simulink model "Perfiles"  (Simulink 8.5)
settings: Solver=ode45  StartTime=0.0  StopTime=tf  RelTol=1e-3
values from neighbouring files (symbols this model uses):
  Kp11 = 238.3924    [EtanolFouriergradiente.m]
  Kp12 = 35.9587    [EtanolFouriergradiente.m]
  Kp1I = 2.7378    [EtanolFouriergradiente.m]
  kp1I = 9.9722    [EtanolFouriergradiente.m]
  Ks1 = 159.7525    [EtanolFouriergradiente.m]
  Ks1I = 94.2332    [EtanolFouriergradiente.m]
  Ks1p1 = 1.3409    [EtanolFouriergradiente.m]
  ks1p1 = 18.6121    [EtanolFouriergradiente.m]
  Ks1p2 = 6.7116    [EtanolFouriergradiente.m]
  ks1p2 = 0.5863    [EtanolFouriergradiente.m]
  Ks2 = 0.0726    [EtanolFouriergradiente.m]
  Ks2I = 9.0048    [EtanolFouriergradiente.m]
  Ks2p1 = 0.9129    [EtanolFouriergradiente.m]
  ks2p1 = 1000    [EtanolFouriergradiente.m]
  Ks2p2 = 0.4310    (= 0.431)    [EtanolFouriergradiente.m]
  ks2p2 = 1.150    (= 1.15)    [EtanolFouriergradiente.m]
  landa = 0.5    [EtanolFouriergradiente.m]
  P10 = 5.3    [EtanolFouriergradiente.m]
  P20 = 0.0001    [EtanolFouriergradiente.m]
  S10 = 8.6    [EtanolFouriergradiente.m]
  S20 = 8.6    [EtanolFouriergradiente.m]
  Sf = 300    [EtanolFouriergradiente.m]
  T0 = 0.01    [EtanolFouriergradiente.m]
  um1 = 1.8823    [EtanolFouriergradiente.m]
  um2 = 1.7098    [EtanolFouriergradiente.m]
  V0 = 1.35    [EtanolFouriergradiente.m]
  vs1p1 = 1.5051    [EtanolFouriergradiente.m]
  vs1p2 = 0.00235    [EtanolFouriergradiente.m]
  vs2p1 = 0.3321    [EtanolFouriergradiente.m]
  vs2p2 = 0.1609    [EtanolFouriergradiente.m]
  X0 = 1.5    [EtanolFouriergradiente.m]
  Yp1s1 = 0.5085    [EtanolFouriergradiente.m]
  Yp1s2 = 0.5098    [EtanolFouriergradiente.m]
  Yp2s1 = 0.5331    [EtanolFouriergradiente.m]
  Yp2s2 = 0.4462    [EtanolFouriergradiente.m]
settings Model: Creator=CECI  LastModifiedBy=User
settings DebuggingCC: SolverPrmCheckMsg=warning  FcnCallInpInsideContextMsg=UseLocalSettings

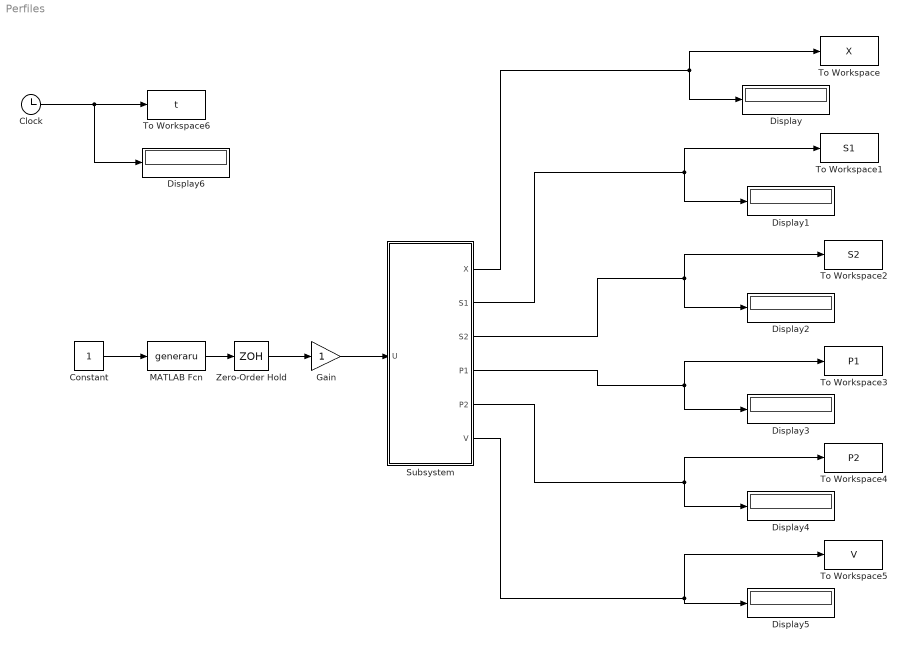
== system Perfiles ==
  Clock : Clock
  Constant : Constant
  Display{,1..6} (7 alike) : Display
  Gain : Gain
  MATLAB Fcn : MATLABFcn  MATLABFcn=generaru  SampleTime=T0
  Subsystem : Subsystem
  To Workspace : ToWorkspace  VariableName=X  SampleTime=T0
  To Workspace1 : ToWorkspace  VariableName=S1  SampleTime=T0
  To Workspace2 : ToWorkspace  VariableName=S2  SampleTime=T0
  To Workspace3 : ToWorkspace  VariableName=P1  SampleTime=T0
  To Workspace4 : ToWorkspace  VariableName=P2  SampleTime=T0
  To Workspace5 : ToWorkspace  VariableName=V  SampleTime=T0
  To Workspace6 : ToWorkspace  VariableName=t  SampleTime=T0
  Zero-Order Hold : ZeroOrderHold  SampleTime=T0
  wires:
  Subsystem/1(X) -> To Workspace/1, Display/1
  Subsystem/2(S1) -> To Workspace1/1, Display1/1
  Clock/1 -> To Workspace6/1, Display6/1
  MATLAB Fcn/1 -> Zero-Order Hold/1
  Constant/1 -> MATLAB Fcn/1
  Zero-Order Hold/1 -> Gain/1
  Gain/1 -> Subsystem/1(U)
  Subsystem/6(V) -> To Workspace5/1, Display5/1
  Subsystem/5(P2) -> Display4/1, To Workspace4/1
  Subsystem/3(S2) -> To Workspace2/1, Display2/1
  Subsystem/4(P1) -> To Workspace3/1, Display3/1

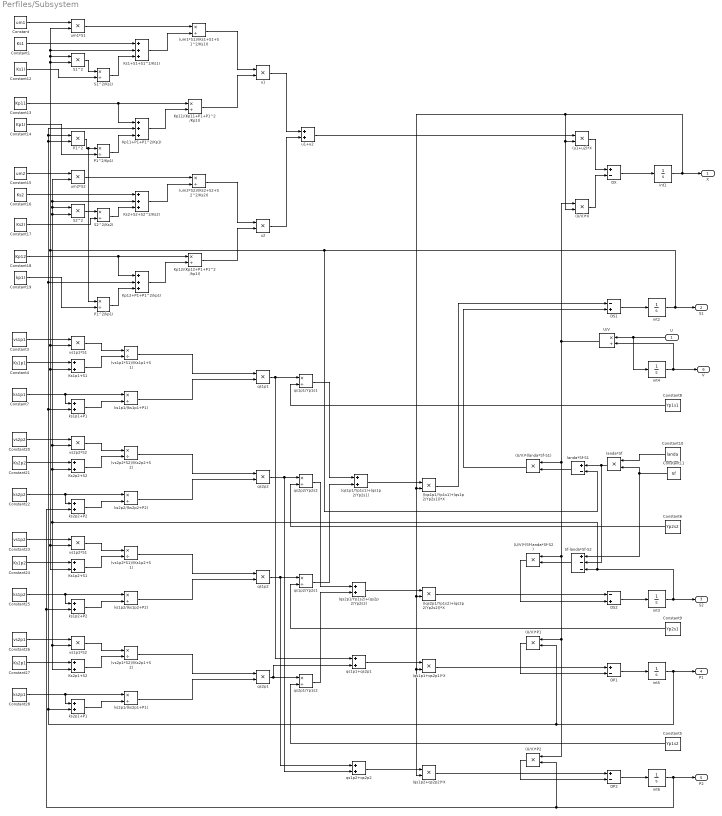
== system Perfiles/Subsystem ==
  U : Inport
  ((qs1p1/Yp1s1)+(qs1p2/Yp2s1))*X : Product  RndMeth=Zero
  ((qs2p1/Yp1s2)+(qs2p2/Yp2s2))*X : Product  RndMeth=Zero
  (U/V)*(Sf-landa*Sf-S2) : Product  RndMeth=Zero
  (U/V)*(landa*Sf-S1) : Product  RndMeth=Zero
  (U/V)*P1 : Product  RndMeth=Zero
  (U/V)*P2 : Product  RndMeth=Zero
  (U/V)*X : Product  RndMeth=Zero
  (qs1p1+qs2p1)*X : Product  RndMeth=Zero
  (qs1p1/Yp1s1)+(qs1p2/Yp2s1) : Sum
  (qs1p2+qs2p2)*X : Product  RndMeth=Zero
  (qs2p1/Yp1s2)+(qs2p2/Yp2s2) : Sum
  (u1+u2)*X : Product  RndMeth=Zero
  (um1*S1)/(Ks1+S1+S1^2/Ks1I) : Product  Inputs=*/
  (um2*S2)/(Ks2+S2+S2^2/Ks2I) : Product  Inputs=*/
  (vs1p1*S1)/(Ks1p1+S1) : Product  Inputs=*/
  (vs1p2*S1)/(Ks1p2+S1) : Product  Inputs=*/
  (vs2p1*S2)/(Ks2p1+S2) : Product  Inputs=*/
  (vs2p2*S2)/(Ks2p2+S2) : Product  Inputs=*/
  Constant : Constant  Value=um1
  Constant1 : Constant  Value=Ks1
  Constant10 : Constant  Value=landa
  Constant11 : Constant  Value=Sf
  Constant12 : Constant  Value=Ks1I
  Constant13 : Constant  Value=Kp11
  Constant14 : Constant  Value=Kp1I
  Constant15 : Constant  Value=um2
  Constant16 : Constant  Value=Ks2
  Constant17 : Constant  Value=Ks2I
  Constant18 : Constant  Value=Kp12
  Constant19 : Constant  Value=kp1I
  Constant20 : Constant  Value=vs2p2
  Constant21 : Constant  Value=Ks2p2
  Constant22 : Constant  Value=ks2p2
  Constant23 : Constant  Value=vs1p2
  Constant24 : Constant  Value=Ks1p2
  Constant25 : Constant  Value=ks1p2
  Constant26 : Constant  Value=vs2p1
  Constant27 : Constant  Value=Ks2p1
  Constant28 : Constant  Value=ks2p1
  Constant3 : Constant  Value=vs1p1
  Constant4 : Constant  Value=Ks1p1
  Constant5 : Constant  Value=Yp1s2
  Constant6 : Constant  Value=Yp2s2
  Constant7 : Constant  Value=ks1p1
  Constant8 : Constant  Value=Yp1s1
  Constant9 : Constant  Value=Yp2s1
  DP1 : Sum  Inputs=+-
  DP2 : Sum  Inputs=+-
  DS1 : Sum  Inputs=-+
  DS2 : Sum  Inputs=-+
  DX : Sum  Inputs=+-
  Kp11+P1+P1^2/Kp1I : Sum  Inputs=+++
  Kp11/(Kp11+P1+P1^2/Kp1I) : Product  Inputs=*/
  Kp12+P1+P1^2/kp1I : Sum  Inputs=+++
  Kp12/(Kp12+P1+P1^2/kp1I) : Product  Inputs=*/
  Ks1+S1+S1^2/Ks1I : Sum  Inputs=+++
  Ks1p1+S1 : Sum
  Ks1p2+S1 : Sum
  Ks2+S2+S2^2/Ks2I : Sum  Inputs=+++
  Ks2p1+S2 : Sum
  Ks2p2+S2 : Sum
  P1^2 : Product  RndMeth=Zero
  P1^2/Kp1I : Product  Inputs=*/
  P1^2/kp1I : Product  Inputs=*/
  S1^2 : Product  RndMeth=Zero
  S1^2/Ks1I : Product  Inputs=*/
  S2^2 : Product  RndMeth=Zero
  S2^2/Ks2I : Product  Inputs=*/
  Sf-landa*Sf-S2 : Sum  Inputs=+--
  U/V : Product  Inputs=*/
  int1 : Integrator  InitialCondition=X0  UpperSaturationLimit=40  LowerSaturationLimit=0
  int2 : Integrator  InitialCondition=S10  UpperSaturationLimit=10  LowerSaturationLimit=0
  int3 : Integrator  InitialCondition=S20  UpperSaturationLimit=100  LowerSaturationLimit=0
  int4 : Integrator  InitialCondition=V0  UpperSaturationLimit=10  LowerSaturationLimit=0
  int5 : Integrator  InitialCondition=P10  UpperSaturationLimit=100  LowerSaturationLimit=0
  int6 : Integrator  InitialCondition=P20  UpperSaturationLimit=100  LowerSaturationLimit=0
  ks1p1+P1 : Sum
  ks1p1/(ks1p1+P1) : Product  Inputs=*/
  ks1p2+P2 : Sum
  ks1p2/(ks1p2+P2) : Product  Inputs=*/
  ks2p1+P1 : Sum
  ks2p1/(ks2p1+P1) : Product  Inputs=*/
  ks2p2+P2 : Sum
  ks2p2/(ks2p2+P2) : Product  Inputs=*/
  landa*Sf : Product  RndMeth=Zero
  landa*Sf-S1 : Sum  Inputs=+-
  qs1p1 : Product  RndMeth=Zero
  qs1p1+qs2p1 : Sum
  qs1p1/Yp1s1 : Product  Inputs=*/
  qs1p2 : Product  RndMeth=Zero
  qs1p2+qs2p2 : Sum
  qs1p2/Yp2s1 : Product  Inputs=*/
  qs2p1 : Product  RndMeth=Zero
  qs2p1/Yp1s2 : Product  Inputs=*/
  qs2p2 : Product  RndMeth=Zero
  qs2p2/Yp2s2 : Product  Inputs=*/
  u1 : Product  RndMeth=Zero
  u1+u2 : Sum
  u2 : Product  RndMeth=Zero
  um1*S1 : Product  RndMeth=Zero
  um2*S2 : Product  RndMeth=Zero
  vs1p1*S1 : Product  RndMeth=Zero
  vs1p1*S2 : Product  RndMeth=Zero
  vs1p2*S1 : Product  RndMeth=Zero
  vs2p2*S2 : Product  RndMeth=Zero
  X : Outport
  S1 : Outport  Port=2
  S2 : Outport  Port=3
  P1 : Outport  Port=4
  P2 : Outport  Port=5
  V : Outport  Port=6
  wires:
  int1/1 -> X/1, (u1+u2)*X/2, (U/V)*X/2, ((qs1p1/Yp1s1)+(qs1p2/Yp2s1))*X/2, ((qs2p1/Yp1s2)+(qs2p2/Yp2s2))*X/2, (qs1p1+qs2p1)*X/2, (qs1p2+qs2p2)*X/2
  Constant/1 -> um1*S1/1
  S1^2/1 -> S1^2/Ks1I/1
  Constant12/1 -> S1^2/Ks1I/2
  Constant1/1 -> Ks1+S1+S1^2/Ks1I/1
  S1^2/Ks1I/1 -> Ks1+S1+S1^2/Ks1I/3
  P1^2/1 -> P1^2/Kp1I/1, P1^2/kp1I/1
  Constant14/1 -> P1^2/Kp1I/2
  P1^2/Kp1I/1 -> Kp11+P1+P1^2/Kp1I/3
  um1*S1/1 -> (um1*S1)/(Ks1+S1+S1^2/Ks1I)/1
  Ks1+S1+S1^2/Ks1I/1 -> (um1*S1)/(Ks1+S1+S1^2/Ks1I)/2
  Constant13/1 -> Kp11+P1+P1^2/Kp1I/1, Kp11/(Kp11+P1+P1^2/Kp1I)/1
  Kp11+P1+P1^2/Kp1I/1 -> Kp11/(Kp11+P1+P1^2/Kp1I)/2
  (um1*S1)/(Ks1+S1+S1^2/Ks1I)/1 -> u1/1
  Kp11/(Kp11+P1+P1^2/Kp1I)/1 -> u1/2
  Constant15/1 -> um2*S2/1
  S2^2/1 -> S2^2/Ks2I/1
  Constant17/1 -> S2^2/Ks2I/2
  Constant16/1 -> Ks2+S2+S2^2/Ks2I/1
  S2^2/Ks2I/1 -> Ks2+S2+S2^2/Ks2I/3
  Constant19/1 -> P1^2/kp1I/2
  P1^2/kp1I/1 -> Kp12+P1+P1^2/kp1I/3
  um2*S2/1 -> (um2*S2)/(Ks2+S2+S2^2/Ks2I)/1
  Ks2+S2+S2^2/Ks2I/1 -> (um2*S2)/(Ks2+S2+S2^2/Ks2I)/2
  Constant18/1 -> Kp12+P1+P1^2/kp1I/1, Kp12/(Kp12+P1+P1^2/kp1I)/1
  Kp12+P1+P1^2/kp1I/1 -> Kp12/(Kp12+P1+P1^2/kp1I)/2
  (um2*S2)/(Ks2+S2+S2^2/Ks2I)/1 -> u2/1
  Kp12/(Kp12+P1+P1^2/kp1I)/1 -> u2/2
  u1/1 -> u1+u2/1
  u2/1 -> u1+u2/2
  u1+u2/1 -> (u1+u2)*X/1
  (u1+u2)*X/1 -> DX/1
  (U/V)*X/1 -> DX/2
  DX/1 -> int1/1
  Constant3/1 -> vs1p1*S1/1
  Constant4/1 -> Ks1p1+S1/1
  vs1p1*S1/1 -> (vs1p1*S1)/(Ks1p1+S1)/1
  Ks1p1+S1/1 -> (vs1p1*S1)/(Ks1p1+S1)/2
  Constant7/1 -> ks1p1+P1/1, ks1p1/(ks1p1+P1)/1
  (vs1p1*S1)/(Ks1p1+S1)/1 -> qs1p1/1
  ks1p1/(ks1p1+P1)/1 -> qs1p1/2
  Constant20/1 -> vs2p2*S2/1
  Constant21/1 -> Ks2p2+S2/1
  vs2p2*S2/1 -> (vs2p2*S2)/(Ks2p2+S2)/1
  Ks2p2+S2/1 -> (vs2p2*S2)/(Ks2p2+S2)/2
  Constant22/1 -> ks2p2+P2/1, ks2p2/(ks2p2+P2)/1
  (vs2p2*S2)/(Ks2p2+S2)/1 -> qs2p2/1
  ks2p2/(ks2p2+P2)/1 -> qs2p2/2
  Constant23/1 -> vs1p2*S1/1
  Constant24/1 -> Ks1p2+S1/1
  vs1p2*S1/1 -> (vs1p2*S1)/(Ks1p2+S1)/1
  Ks1p2+S1/1 -> (vs1p2*S1)/(Ks1p2+S1)/2
  Constant25/1 -> ks1p2+P2/1, ks1p2/(ks1p2+P2)/1
  (vs1p2*S1)/(Ks1p2+S1)/1 -> qs1p2/1
  ks1p2/(ks1p2+P2)/1 -> qs1p2/2
  Constant26/1 -> vs1p1*S2/1
  Constant27/1 -> Ks2p1+S2/1
  vs1p1*S2/1 -> (vs2p1*S2)/(Ks2p1+S2)/1
  Ks2p1+S2/1 -> (vs2p1*S2)/(Ks2p1+S2)/2
  Constant28/1 -> ks2p1+P1/1, ks2p1/(ks2p1+P1)/1
  (vs2p1*S2)/(Ks2p1+S2)/1 -> qs2p1/1
  ks2p1/(ks2p1+P1)/1 -> qs2p1/2
  qs1p1/1 -> qs1p1/Yp1s1/1, qs1p1+qs2p1/1
  Constant8/1 -> qs1p1/Yp1s1/2
  qs1p2/1 -> qs1p2/Yp2s1/1, qs1p2+qs2p2/1
  Constant9/1 -> qs1p2/Yp2s1/2
  Constant6/1 -> qs2p2/Yp2s2/2
  qs2p2/1 -> qs2p2/Yp2s2/1, qs1p2+qs2p2/2
  qs2p1/1 -> qs2p1/Yp1s2/1, qs1p1+qs2p1/2
  Constant5/1 -> qs2p1/Yp1s2/2
  qs1p1/Yp1s1/1 -> (qs1p1/Yp1s1)+(qs1p2/Yp2s1)/1
  qs1p2/Yp2s1/1 -> (qs1p1/Yp1s1)+(qs1p2/Yp2s1)/2
  U/1 -> U/V/1, int4/1
  U/V/1 -> (U/V)*X/1, (U/V)*(landa*Sf-S1)/1, (U/V)*(Sf-landa*Sf-S2)/1, (U/V)*P1/1, (U/V)*P2/1
  (qs1p1/Yp1s1)+(qs1p2/Yp2s1)/1 -> ((qs1p1/Yp1s1)+(qs1p2/Yp2s1))*X/1
  Constant10/1 -> landa*Sf/1
  Constant11/1 -> landa*Sf/2, Sf-landa*Sf-S2/1
  landa*Sf/1 -> landa*Sf-S1/1, Sf-landa*Sf-S2/2
  landa*Sf-S1/1 -> (U/V)*(landa*Sf-S1)/2
  ((qs1p1/Yp1s1)+(qs1p2/Yp2s1))*X/1 -> DS1/1
  (U/V)*(landa*Sf-S1)/1 -> DS1/2
  int2/1 -> S1/1, landa*Sf-S1/2, S1^2/1, um1*S1/2, Ks1+S1+S1^2/Ks1I/2, S1^2/2, vs1p1*S1/2, Ks1p1+S1/2, vs1p2*S1/2, Ks1p2+S1/2
  DS1/1 -> int2/1
  qs2p1/Yp1s2/1 -> (qs2p1/Yp1s2)+(qs2p2/Yp2s2)/2
  qs2p2/Yp2s2/1 -> (qs2p1/Yp1s2)+(qs2p2/Yp2s2)/1
  (qs2p1/Yp1s2)+(qs2p2/Yp2s2)/1 -> ((qs2p1/Yp1s2)+(qs2p2/Yp2s2))*X/1
  Sf-landa*Sf-S2/1 -> (U/V)*(Sf-landa*Sf-S2)/2
  ((qs2p1/Yp1s2)+(qs2p2/Yp2s2))*X/1 -> DS2/1
  (U/V)*(Sf-landa*Sf-S2)/1 -> DS2/2
  int3/1 -> S2/1, Sf-landa*Sf-S2/3, S2^2/1, um2*S2/2, Ks2+S2+S2^2/Ks2I/2, S2^2/2, vs2p2*S2/2, Ks2p2+S2/2, vs1p1*S2/2, Ks2p1+S2/2
  DS2/1 -> int3/1
  qs1p1+qs2p1/1 -> (qs1p1+qs2p1)*X/1
  (qs1p1+qs2p1)*X/1 -> DP1/1
  (U/V)*P1/1 -> DP1/2
  int5/1 -> P1/1, (U/V)*P1/2, ks2p1+P1/2, P1^2/2, P1^2/1, Kp11+P1+P1^2/Kp1I/2, Kp12+P1+P1^2/kp1I/2, ks1p1+P1/2
  DP1/1 -> int5/1
  ks1p1+P1/1 -> ks1p1/(ks1p1+P1)/2
  ks2p1+P1/1 -> ks2p1/(ks2p1+P1)/2
  qs1p2+qs2p2/1 -> (qs1p2+qs2p2)*X/1
  (qs1p2+qs2p2)*X/1 -> DP2/1
  (U/V)*P2/1 -> DP2/2
  DP2/1 -> int6/1
  int6/1 -> P2/1, (U/V)*P2/2, ks2p2+P2/2, ks1p2+P2/2
  int4/1 -> V/1, U/V/2
  ks1p2+P2/1 -> ks1p2/(ks1p2+P2)/2
  ks2p2+P2/1 -> ks2p2/(ks2p2+P2)/2
